simulink model "cloud_throughput_sim"  (R2025a)
settings: Solver=VariableStepAuto  StartTime=0.0  StopTime=20  FixedStep=0.5  RelTol=1e-3
settings Model: Creator=root  LastModifiedBy=root

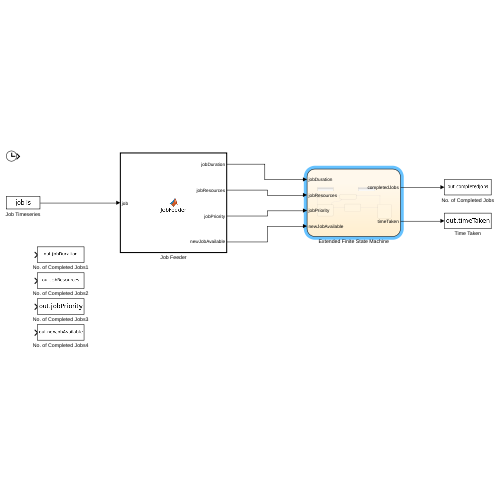
[thumbnail: Simulink's stored preview of the top-level diagram]
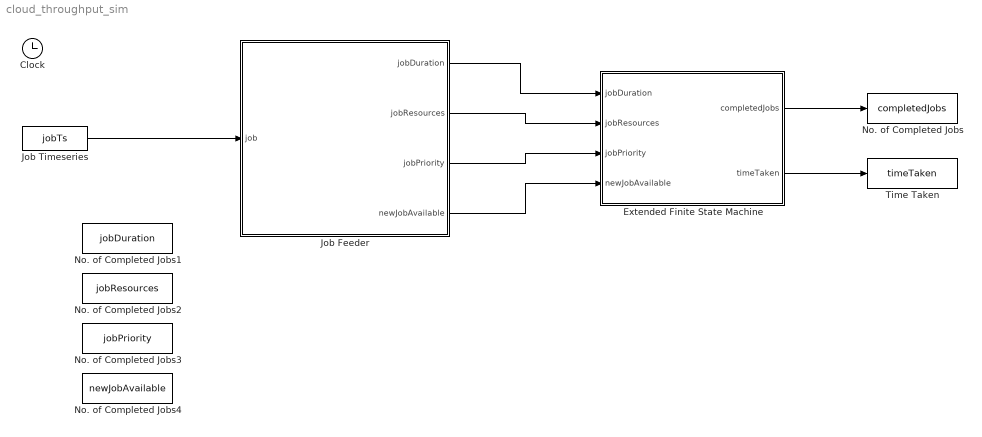
== system cloud_throughput_sim ==
  Clock : Clock
  Extended Finite State Machine : Stateflow chart  TreatAsAtomicUnit=on
  Job Feeder : MATLAB Function  TreatAsAtomicUnit=on
  Job Timeseries : FromWorkspace  VariableName=jobTs  SampleTime=-1  Interpolate=off  OutputAfterFinalValue=Holding final value
  No. of Completed Jobs : ToWorkspace  VariableName=completedJobs  SampleTime=-1
  No. of Completed Jobs1 : ToWorkspace  VariableName=jobDuration  SampleTime=-1
  No. of Completed Jobs2 : ToWorkspace  VariableName=jobResources  SampleTime=-1
  No. of Completed Jobs3 : ToWorkspace  VariableName=jobPriority  SampleTime=-1
  No. of Completed Jobs4 : ToWorkspace  VariableName=newJobAvailable  SampleTime=-1
  Time Taken : ToWorkspace  VariableName=timeTaken  SampleTime=-1
  wires:
  Extended Finite State Machine/1(completedJobs) -> No. of Completed Jobs/1
  Extended Finite State Machine/2(timeTaken) -> Time Taken/1
  Job Timeseries/1 -> Job Feeder/1(job)
  Job Feeder/1(jobDuration) -> Extended Finite State Machine/1(jobDuration)
  Job Feeder/2(jobResources) -> Extended Finite State Machine/2(jobResources)
  Job Feeder/3(jobPriority) -> Extended Finite State Machine/3(jobPriority)
  Job Feeder/4(newJobAvailable) -> Extended Finite State Machine/4(newJobAvailable)

== matlab function cloud_throughput_sim/Job Feeder ==
  data: job input; jobDuration output; jobResources output; jobPriority output; newJobAvailable output
function [jobDuration, jobResources, jobPriority, newJobAvailable] = JobFeeder(job)
% Outputs:
%   jobDuration      - duration of the current job to send to Stateflow
%   jobResources     - requiredResources of the current job
%   jobPriority      - priority of the current job
%   newJobAvailable  - boolean flag indicating if a new job is available this step

persistent lastJob;
if isempty(lastJob)
    lastJob = zeros(3, 1);
end

if lastJob ~= job
    % Output job data to Stateflow
    jobDuration = job(1);
    jobResources = job(2);
    jobPriority = job(3);
    newJobAvailable = true;
    disp([job(1), job(2), job(3)]) % print data to console
else
    jobDuration = 0;
    jobResources = 0;
    jobPriority = 0;
    newJobAvailable = false;
end
lastJob = job;
end

== stateflow chart cloud_throughput_sim/Extended Finite State Machine ==
  state CheckingQueue
    entry:
    [dqJob, dqFound, dqNum] = getNextJobFCFS(availableResources);
    during:
    if newJobAvailable == 1
    enqueueJob(jobDuration, jobResources, jobPriority);
    end
  state Idle
  state SchedulingJob
    entry:
    availableResources = availableResources - currentJobResources;
  state MonitoringJob
    during:
    if newJobAvailable == 1
    enqueueJob(jobDuration, jobResources, jobPriority);
    end
    exit:
    % set outputs
    if dqNum == 0;
    completedJobs = completedJobs + 1;
    else
    completedJobs = completedJobs + dqNum;
    end
    timeTaken = getSimulationTime();
    % reset variables
    availableResources = 8;
    dqFound = 0;
    currentJobDuration = 0;
    currentJobPriority = 0;
    currentJobResources = 0;
    dqJob = [0,0,0];
  state RequestingResources
    entry:
    if dqFound == 1
    currentJobDuration = dqJob(1);
    currentJobResources = dqJob(2);
    currentJobPriority = dqJob(3);
    elseif newJobAvailable == 1
    currentJobDuration = jobDuration;
    currentJobResources = jobResources;
    currentJobPriority = jobPriority;
    end
    during:
    if newJobAvailable == 1
    enqueueJob(jobDuration, jobResources, jobPriority);
    end
  (default) -> Idle
  CheckingQueue -> Idle [order 1] : [dqFound == 0]
  (junction 20) -> CheckingQueue
  MonitoringJob -> (junction 20) : after(currentJobDuration, sec)
  Idle -> RequestingResources : [newJobAvailable == 1]
  CheckingQueue -> RequestingResources [order 2] : [dqFound == 1]
  SchedulingJob -> MonitoringJob
  RequestingResources -> SchedulingJob : [availableResources >= currentJobResources]
  data: duration function_input; requiredResources function_input; priority function_input; availableResources function_input; nextJob function_output; found function_output; numJobs function_output; jobDuration input; jobResources input; jobPriority input; newJobAvailable input; availableResources local =8; currentJobDuration local; currentJobPriority local; currentJobResources local; dqJob local =[0,0,0]; dqFound local =0; dqNum local =0; completedJobs output =0; timeTaken output =0
  function enqueueJob(duration, requiredResources, priority):
    | function enqueueJob(duration, requiredResources, priority)
    |     persistent queue;
    |     if isempty(queue)
    |         queue = zeros(20,3);  % Initialize empty job queue
    |     end
    | 
    |     % Create a new job object
    |     newJob = [duration, requiredResources, priority];
    | 
    |     % Append to the queue
    |     for i = 1:length(queue)
    |        job = queue(i,:);
    |        if job(1) == 0 && job(2) == 0 && job(3) == 0
    |            queue(i,:) = newJob;
    |        end
    |     end
    | end
  function [nextJob, found, numJobs] = getNextJobFCFS(availableResources):
    | function [nextJob, found, numJobs] = getNextJobFCFS(availableResources)
    |     persistent queue
    |     if isempty(queue)
    |         queue = zeros(20,3);
    |     end
    | 
    |     found = 0;
    |     combinedDuration = 0;
    |     combinedResources = 0;
    |     indicesToRemove = [];
    | 
    |     for i = 1:length(queue)
    |         job = queue(i,:);
    |         if job(1) == 0 && job(2) == 0 && job(3) == 0
    |             break;
    |         end
    |         if combinedResources + job(2) <= availableResources
    |             combinedDuration = combinedDuration + job(1);
    |             combinedResources = combinedResources + job(2);
    |             indicesToRemove(end + 1) = i;
    |         else
    |             combinedDuration = job(1);
    |             combinedResources = job(2);
    |             indicesToRemove(1) = i;
    |             break;
    |         end
    |     end
    | 
    |     numJobs = length(indicesToRemove);
    | 
    |     if ~isempty(indicesToRemove)
    |         % Create a combined Job
    |         firstJob = queue(indicesToRemove(1),:);  % Use arrivalTime/priority from first
    |         nextJob = [combinedDuration, combinedResources, firstJob(3)];
    |         % Remove selected jobs from queue (replace with zeros and move
    |         % others to head)
    |         for i = 1:length(indicesToRemove)
    |             queue(i,:) = [0,0,0];
    |         end
    |         % bubble non-zero rows to the top
    |         % Find rows that are NOT [0, 0, 0]
    |         nonZeroRows = any(queue ~= 0, 2);  % Logical index of non-zero rows
    | 
    |         % Extract non-zero rows
    |         nonZeroData = queue(nonZeroRows, :);
    | 
    |         % Count how many non-zero rows
    |         n = size(nonZeroData, 1);
    | 
    |         % Create output array with all zeros
    |         queue = zeros(size(queue));
    | 
    |         % Place non-zero rows at the top
    |         queue(1:n, :) = nonZeroData;
    |         found = 1;
    |     else 
    |         % Nothing fit, return empty/default job
    |         nextJob = [0,0,0];
    |     end
    | end
